simulink model "Stateflow"  (R2017a)
settings: Solver=VariableStepAuto  StartTime=0.0  StopTime=10.0  RelTol=1e-3
undefined symbols (not defined in the file): sigbuilder_block
settings Model: Creator=Owen  LastModifiedBy=Owen

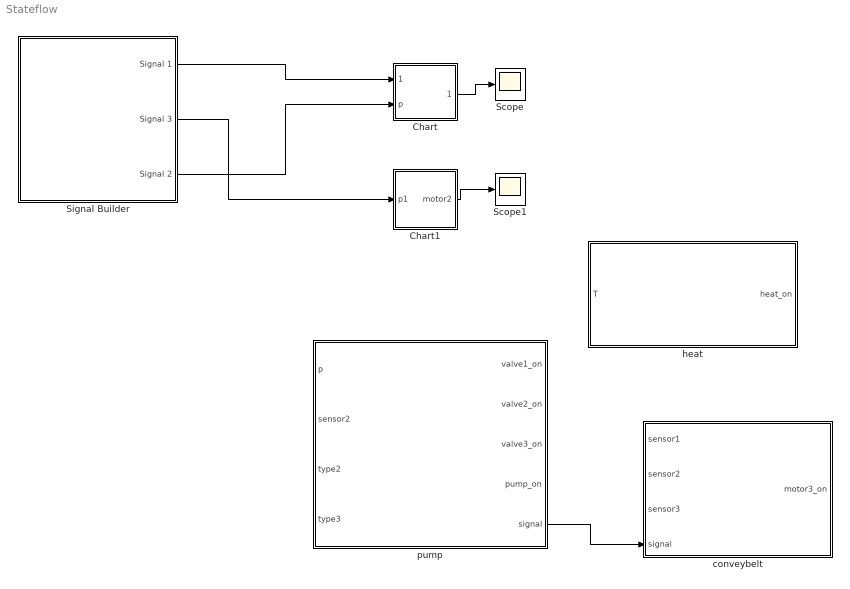
== system Stateflow ==
  Chart : Stateflow chart  TreatAsAtomicUnit=on
  Chart1 : Stateflow chart  TreatAsAtomicUnit=on
  Scope : Scope
  Scope1 : Scope
  Signal Builder : Subsystem  Tag=STV Subsys  LoadFcn=sigbuilder_block('load');  StartFcn=sigbuilder_block('start');  StopFcn=sigbuilder_block('stop');  ClipboardFcn=sigbuilder_block('clipboard');  mask(Sigbuilder block){tuvar=[0:10]}
      mask help: Simulink:masks:SigbuilderBlock_MD
      mask init:
      | if ~strcmp(get_param(bdroot(gcbh),'SimulationStatus'),'stopped') tuvar = sigbuilder_block('maskInit'); end
      settings: CopyFcn=sigbuilder_block('copy');  DeleteFcn=sigbuilder_block('delete');  ModelCloseFcn=sigbuilder_block('modelClose');  PreSaveFcn=sigbuilder_block('preSave');  PauseFcn=sigbuilder_block('pause');  ContinueFcn=sigbuilder_block('continue');  NameChangeFcn=sigbuilder_block('namechange');  OpenFcn=sigbuilder_block('open',[426.75 -123.75 718.5 700.5 ]);  CloseFcn=sigbuilder_block('close');
      mask Display: plot(0, 0, 100, 100,[2, 2, 32, 32, 2], [68, 8, 8, 68, 68],[32, 2], [38, 38], [32, 19, 2],[53, 60, 44], [32, 17, 17, 2],[16, 16, 31, 31]);txt = getActiveGroup(gcbh);text(2, 100, txt,'verticalAlignment', 'top');
  conveybelt : Stateflow chart  TreatAsAtomicUnit=on
  heat : Stateflow chart  TreatAsAtomicUnit=on
  pump : Stateflow chart  TreatAsAtomicUnit=on
  wires:
  Signal Builder/2(Signal 3) -> Chart1/1(p1)
  Signal Builder/3(Signal 2) -> Chart/2(p)
  Chart/1(motor1) -> Scope/1
  Chart1/1(motor2) -> Scope1/1
  Signal Builder/1(Signal 1) -> Chart/1(sensor1)
  pump/5(signal) -> conveybelt/4(signal)

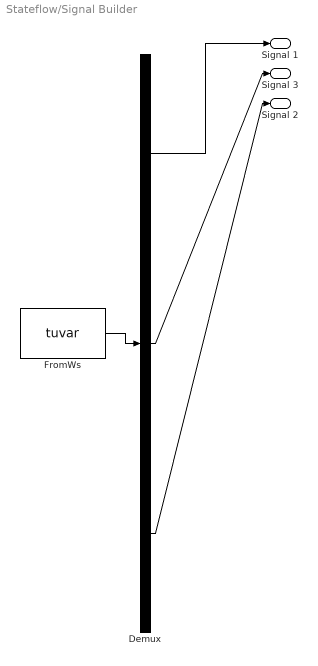
== system Stateflow/Signal Builder ==
  Demux : Demux  Tag=STV Demux  Outputs=3
  FromWs : FromWorkspace  Tag=STV FromWs  VariableName=tuvar  SampleTime=0
      SigBuilderData=|
      | common.afterFinalStr = 'Extrapolate'
      | common.sampleTime = 0
      | dataSet.timeRange = [0 10]
      | dataSet.name = 'Group 1'
      | sbobj.Groups.Name = 'Group 1'
      | sbobj.Groups.Signals(1).Name = 'Signal 1'
      | sbobj.Groups.Signals(1).XData = [0 7 7 10]
      | sbobj.Groups.Signals(1).YData = [0 0 1 1]
      | sbobj.Groups.Signals(2).Name = 'Signal 3'
      | sbobj.Groups.Signals(2).XData = [0 1.01 1.01 10]
      | sbobj.Groups.Signals(2).YData = [1 1 0 0]
      | sbobj.Groups.Signals(3).Name = 'Signal 2'
      | sbobj.Groups.Signals(3).XData = [0 2 2 10]
      | sbobj.Groups.Signals(3).YData = [0 0 1 1]
  Signal 1 : Outport  Tag=STV Outport
  Signal 3 : Outport  Tag=STV Outport  Port=2
  Signal 2 : Outport  Tag=STV Outport  Port=3
  wires:
  Demux/1 -> Signal 1/1
  FromWs/1 -> Demux/1
  Demux/2 -> Signal 3/1
  Demux/3 -> Signal 2/1

== stateflow chart Stateflow/heat ==
  state heatOff
    en:heat_on=0
  state heatOn
    en:heat_on=1
  heatOff -> heatOn : [T<80]
  (default) -> heatOff
  heatOn -> heatOff : [T>99]
  data: T input; heat_on output

== stateflow chart Stateflow/conveybelt ==
  state motor3_off
    en:motor3_on=0
  state motor3_on
    en:motor3_on=1
  motor3_off -> motor3_on [commented out] : [motor3_mode==1]
  motor3_on -> motor3_off : [motor3_mode==0]
  data: sensor1 input; sensor2 input; sensor3 input; signal input; motor3_mode local; motor3_on output
  function motor3_mode:
    | function motor3_mode
    | 
    | aVarTruthTableCondition_1 = false;
    | aVarTruthTableCondition_2 = false;
    | aVarTruthTableCondition_3 = false;
    | aVarTruthTableCondition_4 = false;
    | 
    | 
    | % sensor1
    | 
    | aVarTruthTableCondition_1 = logical(sensor1==1);
    | 
    | % sensor2
    | 
    | aVarTruthTableCondition_2 = logical(sensor2==1);
    | 
    | % signal
    | 
    | aVarTruthTableCondition_3 = logical(signal==1);
    | 
    | % sensor3
    | 
    | aVarTruthTableCondition_4 = logical(sensor3==1);
    | 
    | if (aVarTruthTableCondition_1)
    |     A1();
    | elseif (aVarTruthTableCondition_2 && ~aVarTruthTableCondition_3)
    |     A2();
    | elseif (aVarTruthTableCondition_3)
    |     A1();
    | elseif (aVarTruthTableCondition_4)
    |     A2();
    | else % Default
    |     A2();
    | end
    | 
    | function A1()
    | 
    | % motor3_on
    | 
    | motor3_mode=1
    | 
    | function A2()
    | 
    | % motor3_off
    | 
    | motor3_mode=0

== stateflow chart Stateflow/pump ==
  state valve2control [parallel]
    settings: executionOrder=2
    state valve2_off
      en:valve2_on=0
    state valve2_on
      en:valve2_on=1
    (default) -> valve2_off
    valve2_off -> valve2_on : {[(type2==1||type3==1)&&sensor2==1]}
    valve2_on -> valve2_off : [after(20,sec)]
  state valve1control [parallel]
    settings: executionOrder=1
    state valve1_off
      en:valve1_on=0
    state valve1_on
      en:valve1_on=1
    (default) -> valve1_off
    valve1_off -> valve1_on : {[p==1&&sensor2==1]}
    valve1_on -> valve1_off : [after(30,sec)]
  state valve3control [parallel]
    settings: executionOrder=4
    state valve3_off
      en:valve3_on=0
    state valve3_on
      en:valve3_on=1
    (default) -> valve3_off
    valve3_off -> valve3_on : {[type3==1&&sensor2==1]}
    valve3_on -> valve3_off : [after(10,sec)]
  state pumpcontrol [parallel]
    settings: executionOrder=3
    state pump_off
      en:pump_on=0
    state pump_on
      en:pump_on=1
    state signal
      en:signal=1
    (default) -> pump_off
    pump_off -> pump_on : {[p==1&&sensor2==1]}
    signal -> pump_off
    pump_on -> signal : [after(100,sec)]
  data: p input; sensor2 input; type2 input; type3 input; valve1_on output; valve2_on output; valve3_on output; pump_on output; signal output

== stateflow chart Stateflow/Chart ==
  state motor1_on
    entry: motor1=1
  state motor1_off
    entry: motor1=0
  motor1_on -> motor1_off : [sensor1==1]
  (default) -> motor1_off
  motor1_off -> motor1_on : [sensor1==0&&p==1]
  data: sensor1 input; p input; motor1 output

== stateflow chart Stateflow/Chart1 ==
  state motor2_down
    entry: motor2=-1
  state motor2_stop
    entry: motor2=0
  state motor2_up
    entry: motor2=1
  motor2_down -> motor2_stop : after(5,sec)
  (default) -> motor2_stop
  motor2_stop -> motor2_down [order 2] : after(1,sec)
  motor2_stop -> motor2_up [order 1] : [p1==1]
  motor2_up -> motor2_stop : after(1,sec)
  data: p1 input; motor2 output
